simulink model "radians_to_torque"  (R2024a)
settings: Solver=VariableStepAuto  StartTime=0.0  StopTime=10.0  RelTol=1e-3
settings Model: Creator=robertbergbaum  LastModifiedBy=robertbergbaum

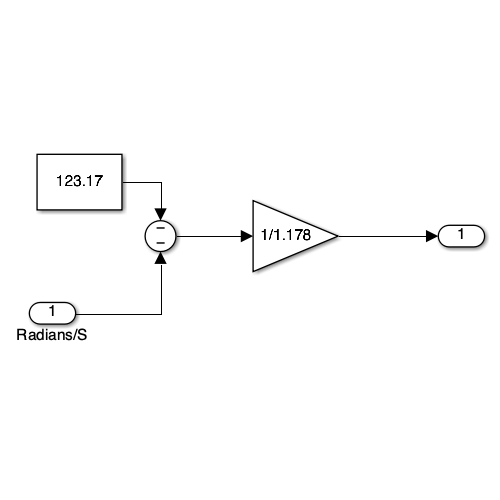
[thumbnail: Simulink's stored preview of the top-level diagram]
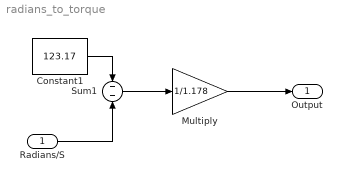
== system radians_to_torque ==
  Radians/S : Inport
  Constant1 : Constant  Value=123.17
  Multiply : Gain  Gain=1/1.178
  Sum1 : Sum  Inputs=--
  Output : Outport
  wires:
  Constant1/1 -> Sum1/1
  Radians/S/1 -> Sum1/2
  Sum1/1 -> Multiply/1
  Multiply/1 -> Output/1
